simulink model "QuadrotorSimulink"  (Simulink 7.2)
settings: Solver=ode45  StartTime=0.0  StopTime=10  RelTol=1e-3
undefined symbols (not defined in the file or in its folder): Quad
settings Model: Creator=test  LastModifiedBy=test

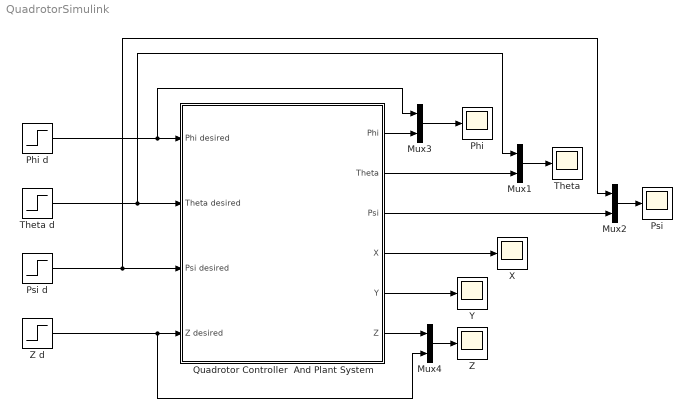
== system QuadrotorSimulink ==
  Mux{1..4} (4 alike) : Mux  Inputs=2
  Phi : Scope
  Phi d : Step  After=0  SampleTime=0
  Psi : Scope
      settings: SaveName=ScopeData2
  Psi d : Step  After=0  SampleTime=0
  Quadrotor Controller  And Plant System : Subsystem
  Theta : Scope
  Theta d : Step  After=0  SampleTime=0
  X : Scope
      settings: SaveName=ScopeData5
  Y : Scope
      settings: SaveName=ScopeData4
  Z : Scope
      settings: SaveName=ScopeData3
  Z d : Step  After=-1  SampleTime=0
  wires:
  Phi d/1 -> Quadrotor Controller  And Plant System/1(Phi desired), Mux3/1
  Theta d/1 -> Quadrotor Controller  And Plant System/2(Theta desired), Mux1/1
  Psi d/1 -> Quadrotor Controller  And Plant System/3(Psi desired), Mux2/1
  Z d/1 -> Quadrotor Controller  And Plant System/4(Z desired), Mux4/2
  Quadrotor Controller  And Plant System/1(Phi) -> Mux3/2
  Mux3/1 -> Phi/1
  Mux1/1 -> Theta/1
  Mux2/1 -> Psi/1
  Quadrotor Controller  And Plant System/2(Theta) -> Mux1/2
  Quadrotor Controller  And Plant System/3(Psi) -> Mux2/2
  Mux4/1 -> Z/1
  Quadrotor Controller  And Plant System/6(Z) -> Mux4/1
  Quadrotor Controller  And Plant System/5(Y) -> Y/1
  Quadrotor Controller  And Plant System/4(X) -> X/1

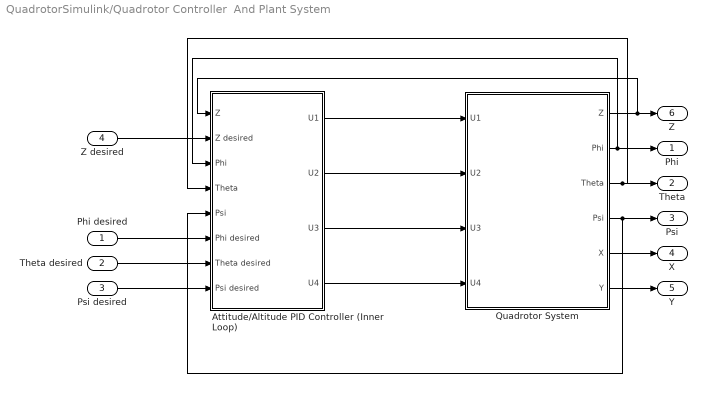
== system QuadrotorSimulink/Quadrotor Controller  And Plant System ==
  Phi desired : Inport  OutDataType=fixdt(1, 16)  OutScaling=2^0
  Theta desired : Inport  Port=2  OutDataType=fixdt(1, 16)  OutScaling=2^0
  Psi desired : Inport  Port=3  OutDataType=fixdt(1, 16)  OutScaling=2^0
  Z desired : Inport  Port=4  OutDataType=fixdt(1, 16)  OutScaling=2^0
  Attitude/Altitude PID Controller (Inner Loop) : Subsystem
  Quadrotor System : Subsystem
  Phi : Outport  OutDataType=fixdt(1, 16)  OutScaling=2^0
  Theta : Outport  Port=2  OutDataType=fixdt(1, 16)  OutScaling=2^0
  Psi : Outport  Port=3  OutDataType=fixdt(1, 16)  OutScaling=2^0
  X : Outport  Port=4  OutDataType=fixdt(1, 16)  OutScaling=2^0
  Y : Outport  Port=5  OutDataType=fixdt(1, 16)  OutScaling=2^0
  Z : Outport  Port=6  OutDataType=fixdt(1, 16)  OutScaling=2^0
  wires:
  Attitude/Altitude PID Controller (Inner Loop)/2(U2) -> Quadrotor System/2(U2)
  Psi desired/1 -> Attitude/Altitude PID Controller (Inner Loop)/8(Psi desired)
  Z desired/1 -> Attitude/Altitude PID Controller (Inner Loop)/2(Z desired)
  Attitude/Altitude PID Controller (Inner Loop)/3(U3) -> Quadrotor System/3(U3)
  Theta desired/1 -> Attitude/Altitude PID Controller (Inner Loop)/7(Theta desired)
  Phi desired/1 -> Attitude/Altitude PID Controller (Inner Loop)/6(Phi desired)
  Quadrotor System/2(Phi) -> Attitude/Altitude PID Controller (Inner Loop)/3(Phi), Phi/1
  Quadrotor System/3(Theta) -> Attitude/Altitude PID Controller (Inner Loop)/4(Theta), Theta/1
  Quadrotor System/4(Psi) -> Attitude/Altitude PID Controller (Inner Loop)/5(Psi), Psi/1
  Quadrotor System/5(X) -> X/1
  Quadrotor System/6(Y) -> Y/1
  Quadrotor System/1(Z) -> Z/1, Attitude/Altitude PID Controller (Inner Loop)/1(Z)
  Attitude/Altitude PID Controller (Inner Loop)/4(U4) -> Quadrotor System/4(U4)
  Attitude/Altitude PID Controller (Inner Loop)/1(U1) -> Quadrotor System/1(U1)

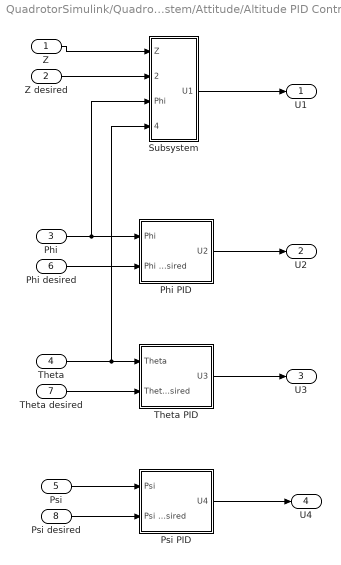
== system QuadrotorSimulink/Quadrotor Controller  And Plant System/Attitude/Altitude PID Controller (Inner Loop) ==
  Z : Inport  OutDataType=fixdt(1, 16)  OutScaling=2^0
  Z desired : Inport  Port=2  OutDataType=fixdt(1, 16)  OutScaling=2^0
  Phi : Inport  Port=3  OutDataType=fixdt(1, 16)  OutScaling=2^0
  Theta : Inport  Port=4  OutDataType=fixdt(1, 16)  OutScaling=2^0
  Psi : Inport  Port=5  OutDataType=fixdt(1, 16)  OutScaling=2^0
  Phi desired : Inport  Port=6  OutDataType=fixdt(1, 16)  OutScaling=2^0
  Theta desired : Inport  Port=7  OutDataType=fixdt(1, 16)  OutScaling=2^0
  Psi desired : Inport  Port=8  OutDataType=fixdt(1, 16)  OutScaling=2^0
  Phi PID : Subsystem
  Psi PID : Subsystem
  Subsystem : Subsystem
  Theta PID : Subsystem
  U1 : Outport  OutDataType=fixdt(1, 16)  OutScaling=2^0
  U2 : Outport  Port=2  OutDataType=fixdt(1, 16)  OutScaling=2^0
  U3 : Outport  Port=3  OutDataType=fixdt(1, 16)  OutScaling=2^0
  U4 : Outport  Port=4  OutDataType=fixdt(1, 16)  OutScaling=2^0
  wires:
  Subsystem/1(U1) -> U1/1
  Z desired/1 -> Subsystem/2(Z desired)
  Z/1 -> Subsystem/1(Z)
  Phi PID/1(U2) -> U2/1
  Phi desired/1 -> Phi PID/2(Phi desired)
  Phi/1 -> Phi PID/1(Phi), Subsystem/3(Phi)
  Psi PID/1(U4) -> U4/1
  Psi desired/1 -> Psi PID/2(Psi desired)
  Psi/1 -> Psi PID/1(Psi)
  Theta PID/1(U3) -> U3/1
  Theta desired/1 -> Theta PID/2(Theta desired)
  Theta/1 -> Theta PID/1(Theta), Subsystem/4(Theta)

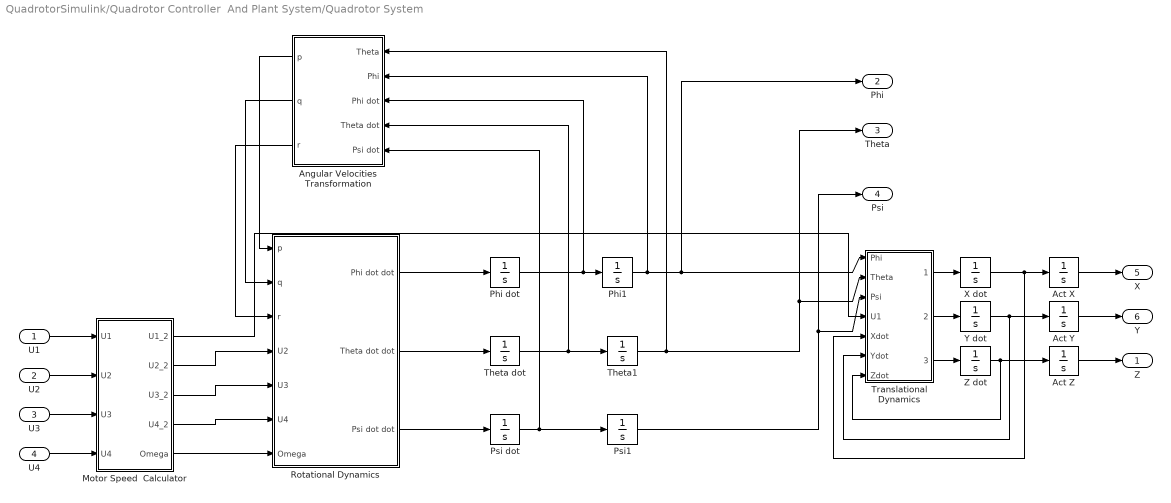
== system QuadrotorSimulink/Quadrotor Controller  And Plant System/Quadrotor System ==
  U1 : Inport  OutDataType=fixdt(1, 16)  OutScaling=2^0
  U2 : Inport  Port=2  OutDataType=fixdt(1, 16)  OutScaling=2^0
  U3 : Inport  Port=3  OutDataType=fixdt(1, 16)  OutScaling=2^0
  U4 : Inport  Port=4  OutDataType=fixdt(1, 16)  OutScaling=2^0
  Act X : Integrator
  Act Y : Integrator
  Act Z : Integrator
  Angular Velocities Transformation : Subsystem  Orientation=left
  Motor Speed  Calculator : Subsystem
  Phi dot : Integrator
  Phi1 : Integrator  ZeroCross=off
  Psi dot : Integrator  ZeroCross=off
  Psi1 : Integrator  ZeroCross=off
  Rotational Dynamics : Subsystem
  Theta dot : Integrator  ZeroCross=off
  Theta1 : Integrator  ZeroCross=off
  Translational Dynamics : Subsystem
  X dot : Integrator
  Y dot : Integrator
  Z dot : Integrator
  Z : Outport  OutDataType=fixdt(1, 16)  OutScaling=2^0
  Phi : Outport  Port=2  OutDataType=fixdt(1, 16)  OutScaling=2^0
  Theta : Outport  Port=3  OutDataType=fixdt(1, 16)  OutScaling=2^0
  Psi : Outport  Port=4  OutDataType=fixdt(1, 16)  OutScaling=2^0
  X : Outport  Port=5  OutDataType=fixdt(1, 16)  OutScaling=2^0
  Y : Outport  Port=6  OutDataType=fixdt(1, 16)  OutScaling=2^0
  wires:
  Rotational Dynamics/2(Theta dot dot) -> Theta dot/1
  Motor Speed  Calculator/5(Omega) -> Rotational Dynamics/7(Omega)
  Phi1/1 -> Translational Dynamics/1(Phi), Phi/1, Angular Velocities Transformation/2(Phi)
  Theta1/1 -> Translational Dynamics/2(Theta), Theta/1, Angular Velocities Transformation/1(Theta)
  Psi1/1 -> Translational Dynamics/3(Psi), Psi/1
  Translational Dynamics/1(x dotdot) -> X dot/1
  X dot/1 -> Act X/1, Translational Dynamics/5(Xdot)
  Y dot/1 -> Act Y/1, Translational Dynamics/6(Ydot)
  Translational Dynamics/2(y dotdot) -> Y dot/1
  Z dot/1 -> Translational Dynamics/7(Zdot), Act Z/1
  Translational Dynamics/3(z dotdot) -> Z dot/1
  Act X/1 -> X/1
  Act Y/1 -> Y/1
  Act Z/1 -> Z/1
  Psi dot/1 -> Psi1/1, Angular Velocities Transformation/5(Psi dot)
  Theta dot/1 -> Theta1/1, Angular Velocities Transformation/4(Theta dot)
  Phi dot/1 -> Phi1/1, Angular Velocities Transformation/3(Phi dot)
  Rotational Dynamics/3(Psi dot dot) -> Psi dot/1
  Rotational Dynamics/1(Phi dot dot) -> Phi dot/1
  U4/1 -> Motor Speed  Calculator/4(U4)
  U2/1 -> Motor Speed  Calculator/2(U2)
  U3/1 -> Motor Speed  Calculator/3(U3)
  Motor Speed  Calculator/2(U2_2) -> Rotational Dynamics/4(U2)
  Motor Speed  Calculator/3(U3_2) -> Rotational Dynamics/5(U3)
  Motor Speed  Calculator/1(U1_2) -> Translational Dynamics/4(U1)
  U1/1 -> Motor Speed  Calculator/1(U1)
  Motor Speed  Calculator/4(U4_2) -> Rotational Dynamics/6(U4)
  Angular Velocities Transformation/1(p) -> Rotational Dynamics/1(p)
  Angular Velocities Transformation/2(q) -> Rotational Dynamics/2(q)
  Angular Velocities Transformation/3(r) -> Rotational Dynamics/3(r)

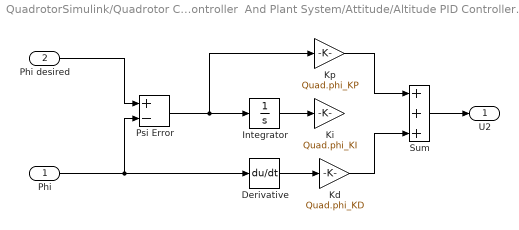
== system QuadrotorSimulink/Quadrotor Controller  And Plant System/Attitude/Altitude PID Controller (Inner Loop)/Phi PID ==
  Phi : Inport  OutDataType=fixdt(1, 16)  OutScaling=2^0
  Phi desired : Inport  Port=2  OutDataType=fixdt(1, 16)  OutScaling=2^0
  Derivative : Derivative
  Integrator : Integrator
  Kd : Gain  Gain=Quad.phi_KD  ParameterDataType=fixdt(1, 16)  ParameterScaling=2^0  OutDataType=fixdt(1, 16)  OutScaling=2^0
  Ki : Gain  Gain=Quad.phi_KI  ParameterDataType=fixdt(1, 16)  ParameterScaling=2^0  OutDataType=fixdt(1, 16)  OutScaling=2^0
  Kp : Gain  Gain=Quad.phi_KP  ParameterDataType=fixdt(1, 16)  ParameterScaling=2^0  OutDataType=fixdt(1, 16)  OutScaling=2^0
  Psi Error : Sum  Inputs=+-  OutDataType=fixdt(1, 16)  OutScaling=2^-10
  Sum : Sum  Inputs=+++  OutDataType=fixdt(1, 16)  OutScaling=2^-10
  U2 : Outport  OutDataType=fixdt(1, 16)  OutScaling=2^0
  wires:
  Phi/1 -> Psi Error/2, Derivative/1
  Phi desired/1 -> Psi Error/1
  Derivative/1 -> Kd/1
  Kp/1 -> Sum/1
  Sum/1 -> U2/1
  Psi Error/1 -> Integrator/1, Kp/1
  Integrator/1 -> Ki/1
  Kd/1 -> Sum/3

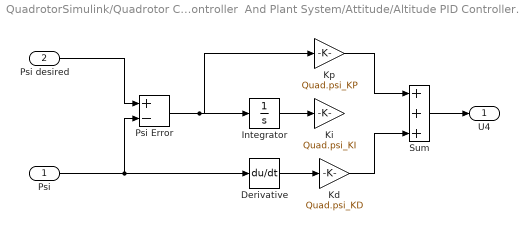
== system QuadrotorSimulink/Quadrotor Controller  And Plant System/Attitude/Altitude PID Controller (Inner Loop)/Psi PID ==
  Psi : Inport  OutDataType=fixdt(1, 16)  OutScaling=2^0
  Psi desired : Inport  Port=2  OutDataType=fixdt(1, 16)  OutScaling=2^0
  Derivative : Derivative
  Integrator : Integrator
  Kd : Gain  Gain=Quad.psi_KD  ParameterDataType=fixdt(1, 16)  ParameterScaling=2^0  OutDataType=fixdt(1, 16)  OutScaling=2^0
  Ki : Gain  Gain=Quad.psi_KI  ParameterDataType=fixdt(1, 16)  ParameterScaling=2^0  OutDataType=fixdt(1, 16)  OutScaling=2^0
  Kp : Gain  Gain=Quad.psi_KP  ParameterDataType=fixdt(1, 16)  ParameterScaling=2^0  OutDataType=fixdt(1, 16)  OutScaling=2^0
  Psi Error : Sum  Inputs=+-  OutDataType=fixdt(1, 16)  OutScaling=2^-10
  Sum : Sum  Inputs=+++  OutDataType=fixdt(1, 16)  OutScaling=2^-10
  U4 : Outport  OutDataType=fixdt(1, 16)  OutScaling=2^0
  wires:
  Psi/1 -> Psi Error/2, Derivative/1
  Psi desired/1 -> Psi Error/1
  Derivative/1 -> Kd/1
  Kp/1 -> Sum/1
  Sum/1 -> U4/1
  Psi Error/1 -> Integrator/1, Kp/1
  Integrator/1 -> Ki/1
  Kd/1 -> Sum/3

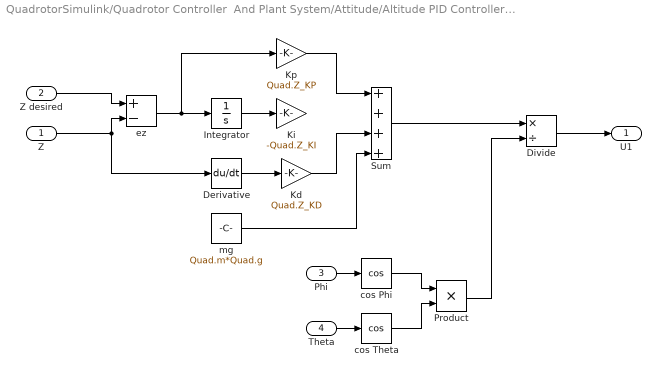
== system QuadrotorSimulink/Quadrotor Controller  And Plant System/Attitude/Altitude PID Controller (Inner Loop)/Subsystem ==
  Z : Inport  OutDataType=fixdt(1, 16)  OutScaling=2^0
  Z desired : Inport  Port=2  OutDataType=fixdt(1, 16)  OutScaling=2^0
  Phi : Inport  Port=3
  Theta : Inport  Port=4
  Derivative : Derivative
  Divide : Product  Inputs=*/  OutDataType=fixdt(1, 16)  OutScaling=2^-10
  Integrator : Integrator
  Kd : Gain  Gain=Quad.Z_KD  ParameterDataType=fixdt(1, 16)  ParameterScaling=2^0  OutDataType=fixdt(1, 16)  OutScaling=2^0
  Ki : Gain  Gain=-Quad.Z_KI  ParameterDataType=fixdt(1, 16)  ParameterScaling=2^0  OutDataType=fixdt(1, 16)  OutScaling=2^0
  Kp : Gain  Gain=Quad.Z_KP  ParameterDataType=fixdt(1, 16)  ParameterScaling=2^0  OutDataType=fixdt(1, 16)  OutScaling=2^0
  Product : Product  OutDataType=fixdt(1, 16)  OutScaling=2^0  RndMeth=Zero
  Sum : Sum  Inputs=++++  OutDataType=fixdt(1, 16)  OutScaling=2^-10
  cos Phi : Trigonometry  Operator=cos
  cos Theta : Trigonometry  Operator=cos
  ez : Sum  Inputs=+-  OutDataType=fixdt(1, 16)  OutScaling=2^-10
  mg : Constant  Value=Quad.m*Quad.g  OutDataType=fixdt(1, 16)  OutScaling=2^0
  U1 : Outport  OutDataType=fixdt(1, 16)  OutScaling=2^0
  wires:
  Z desired/1 -> ez/1
  cos Phi/1 -> Product/1
  cos Theta/1 -> Product/2
  Product/1 -> Divide/2
  Phi/1 -> cos Phi/1
  Theta/1 -> cos Theta/1
  Z/1 -> ez/2, Derivative/1
  Derivative/1 -> Kd/1
  Kp/1 -> Sum/1
  Integrator/1 -> Ki/1
  ez/1 -> Integrator/1, Kp/1
  Sum/1 -> Divide/1
  Divide/1 -> U1/1
  mg/1 -> Sum/4
  Kd/1 -> Sum/3

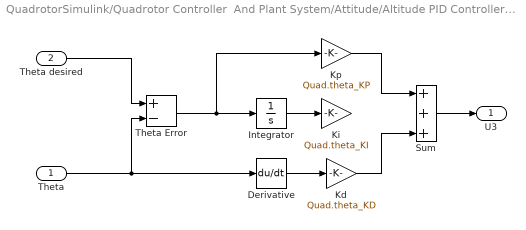
== system QuadrotorSimulink/Quadrotor Controller  And Plant System/Attitude/Altitude PID Controller (Inner Loop)/Theta PID ==
  Theta : Inport  OutDataType=fixdt(1, 16)  OutScaling=2^0
  Theta desired : Inport  Port=2  OutDataType=fixdt(1, 16)  OutScaling=2^0
  Derivative : Derivative
  Integrator : Integrator
  Kd : Gain  Gain=Quad.theta_KD  ParameterDataType=fixdt(1, 16)  ParameterScaling=2^0  OutDataType=fixdt(1, 16)  OutScaling=2^0
  Ki : Gain  Gain=Quad.theta_KI  ParameterDataType=fixdt(1, 16)  ParameterScaling=2^0  OutDataType=fixdt(1, 16)  OutScaling=2^0
  Kp : Gain  Gain=Quad.theta_KP  ParameterDataType=fixdt(1, 16)  ParameterScaling=2^0  OutDataType=fixdt(1, 16)  OutScaling=2^0
  Sum : Sum  Inputs=+++  OutDataType=fixdt(1, 16)  OutScaling=2^-10
  Theta Error : Sum  Inputs=+-  OutDataType=fixdt(1, 16)  OutScaling=2^-10
  U3 : Outport  OutDataType=fixdt(1, 16)  OutScaling=2^0
  wires:
  Theta/1 -> Theta Error/2, Derivative/1
  Theta desired/1 -> Theta Error/1
  Derivative/1 -> Kd/1
  Kp/1 -> Sum/1
  Sum/1 -> U3/1
  Theta Error/1 -> Integrator/1, Kp/1
  Integrator/1 -> Ki/1
  Kd/1 -> Sum/3

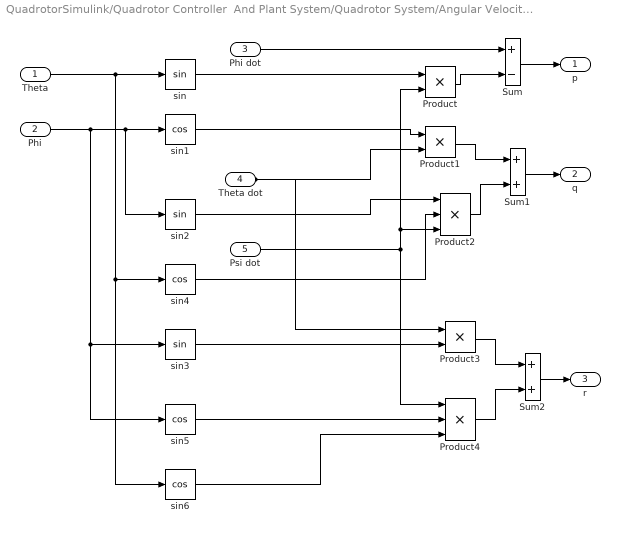
== system QuadrotorSimulink/Quadrotor Controller  And Plant System/Quadrotor System/Angular Velocities Transformation ==
  Theta : Inport  OutDataType=sfix(16)  OutScaling=2^0
  Phi : Inport  Port=2  OutDataType=sfix(16)  OutScaling=2^0
  Phi dot : Inport  Port=3  OutDataType=sfix(16)  OutScaling=2^0
  Theta dot : Inport  Port=4  OutDataType=sfix(16)  OutScaling=2^0
  Psi dot : Inport  Port=5  OutDataType=sfix(16)  OutScaling=2^0
  Product : Product  OutDataType=sfix(16)  OutScaling=2^0  RndMeth=Zero
  Product1 : Product  OutDataType=sfix(16)  OutScaling=2^0  RndMeth=Zero
  Product2 : Product  Inputs=3  OutDataType=sfix(16)  OutScaling=2^0  RndMeth=Zero
  Product3 : Product  OutDataType=sfix(16)  OutScaling=2^0  RndMeth=Zero
  Product4 : Product  Inputs=3  OutDataType=sfix(16)  OutScaling=2^0  RndMeth=Zero
  Sum : Sum  Inputs=+-  OutDataType=sfix(16)  OutScaling=2^0
  Sum1 : Sum  OutDataType=sfix(16)  OutScaling=2^0
  Sum2 : Sum  OutDataType=sfix(16)  OutScaling=2^0
  sin : Trigonometry
  sin{1,4..6} (4 alike) : Trigonometry  Operator=cos
  sin2 : Trigonometry
  sin3 : Trigonometry
  p : Outport  OutDataType=sfix(16)  OutScaling=2^0
  q : Outport  Port=2  OutDataType=sfix(16)  OutScaling=2^0
  r : Outport  Port=3  OutDataType=sfix(16)  OutScaling=2^0
  wires:
  Phi dot/1 -> Sum/1
  Theta/1 -> sin4/1, sin6/1, sin/1
  sin/1 -> Product/1
  Psi dot/1 -> Product/2, Product2/3, Product4/1
  Product/1 -> Sum/2
  Sum/1 -> p/1
  Phi/1 -> sin1/1, sin2/1, sin3/1, sin5/1
  sin1/1 -> Product1/1
  Theta dot/1 -> Product1/2, Product3/1
  Product1/1 -> Sum1/1
  sin2/1 -> Product2/1
  sin4/1 -> Product2/2
  Product2/1 -> Sum1/2
  Sum1/1 -> q/1
  sin3/1 -> Product3/2
  sin5/1 -> Product4/2
  sin6/1 -> Product4/3
  Product3/1 -> Sum2/1
  Product4/1 -> Sum2/2
  Sum2/1 -> r/1

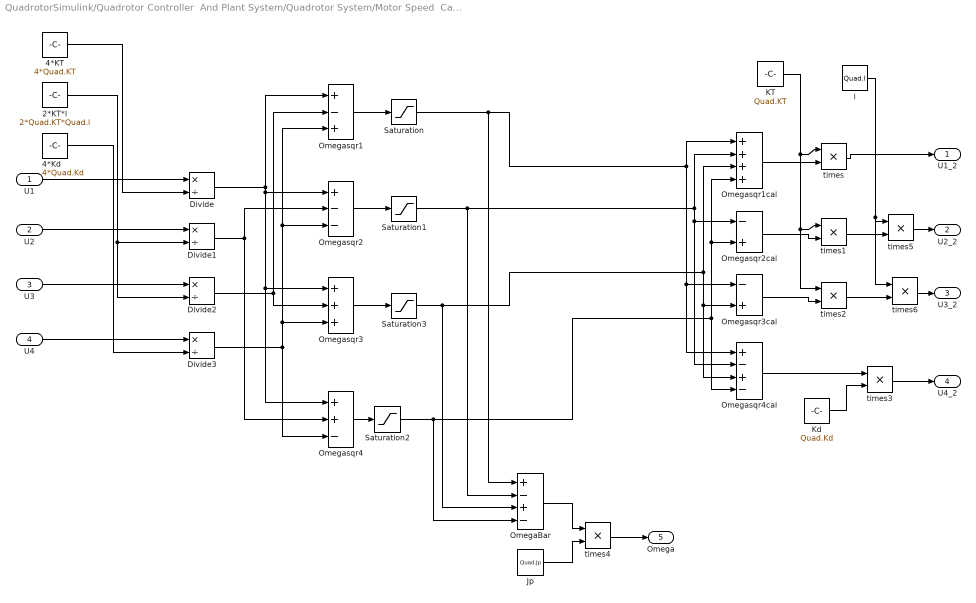
== system QuadrotorSimulink/Quadrotor Controller  And Plant System/Quadrotor System/Motor Speed  Calculator ==
  U1 : Inport  OutDataType=fixdt(1, 16)  OutScaling=2^0
  U2 : Inport  Port=2  OutDataType=fixdt(1, 16)  OutScaling=2^0
  U3 : Inport  Port=3  OutDataType=fixdt(1, 16)  OutScaling=2^0
  U4 : Inport  Port=4  OutDataType=fixdt(1, 16)  OutScaling=2^0
  2*KT*l : Constant  Value=2*Quad.KT*Quad.l  OutDataType=fixdt(1, 16)  OutScaling=2^0
  4*KT : Constant  Value=4*Quad.KT  OutDataType=fixdt(1, 16)  OutScaling=2^0
  4*Kd : Constant  Value=4*Quad.Kd  OutDataType=fixdt(1, 16)  OutScaling=2^0
  Divide{,1..3} (4 alike) : Product  Inputs=*/  OutDataType=fixdt(1, 16)  OutScaling=2^-10
  Jp : Constant  Value=Quad.Jp  OutDataType=fixdt(1, 16)  OutScaling=2^0
  KT : Constant  Value=Quad.KT  OutDataType=fixdt(1, 16)  OutScaling=2^0
  Kd : Constant  Value=Quad.Kd  OutDataType=fixdt(1, 16)  OutScaling=2^0
  OmegaBar : Sum  Inputs=+-+-  OutDataType=fixdt(1, 16)  OutScaling=2^-10
  Omegasqr1 : Sum  Inputs=+-+  OutDataType=fixdt(1, 16)  OutScaling=2^-10
  Omegasqr1cal : Sum  Inputs=++++  OutDataType=fixdt(1, 16)  OutScaling=2^-10
  Omegasqr2 : Sum  Inputs=+--  OutDataType=fixdt(1, 16)  OutScaling=2^-10
  Omegasqr2cal : Sum  Inputs=-+  OutDataType=fixdt(1, 16)  OutScaling=2^-10
  Omegasqr3 : Sum  Inputs=+++  OutDataType=fixdt(1, 16)  OutScaling=2^-10
  Omegasqr3cal : Sum  Inputs=-+  OutDataType=fixdt(1, 16)  OutScaling=2^-10
  Omegasqr4 : Sum  Inputs=++-  OutDataType=fixdt(1, 16)  OutScaling=2^-10
  Omegasqr4cal : Sum  Inputs=+-+-  OutDataType=fixdt(1, 16)  OutScaling=2^-10
  Saturation{,1..3} (4 alike) : Saturate  UpperLimit=Quad.max_motor_speed  LowerLimit=Quad.min_motor_speed  OutDataType=sfix(16)  OutScaling=2^0
  l : Constant  Value=Quad.l  OutDataType=fixdt(1, 16)  OutScaling=2^0
  times{,1..6} (7 alike) : Product  Inputs=**  OutDataType=fixdt(1, 16)  OutScaling=2^-10
  U1_2 : Outport  OutDataType=fixdt(1, 16)  OutScaling=2^0
  U2_2 : Outport  Port=2  OutDataType=fixdt(1, 16)  OutScaling=2^0
  U3_2 : Outport  Port=3  OutDataType=fixdt(1, 16)  OutScaling=2^0
  U4_2 : Outport  Port=4  OutDataType=fixdt(1, 16)  OutScaling=2^0
  Omega : Outport  Port=5  OutDataType=fixdt(1, 16)  OutScaling=2^0
  wires:
  U1/1 -> Divide/1
  4*KT/1 -> Divide/2
  U2/1 -> Divide1/1
  2*KT*l/1 -> Divide1/2, Divide2/2
  U3/1 -> Divide2/1
  U4/1 -> Divide3/1
  4*Kd/1 -> Divide3/2
  Divide/1 -> Omegasqr1/1, Omegasqr2/1, Omegasqr3/1, Omegasqr4/1
  Divide2/1 -> Omegasqr1/2, Omegasqr3/2
  Divide3/1 -> Omegasqr1/3, Omegasqr2/3, Omegasqr3/3, Omegasqr4/3
  Divide1/1 -> Omegasqr2/2, Omegasqr4/2
  OmegaBar/1 -> times4/1
  times4/1 -> Omega/1
  KT/1 -> times/1, times1/1, times2/1
  Omegasqr1cal/1 -> times/2
  Omegasqr2cal/1 -> times1/2
  Omegasqr3cal/1 -> times2/2
  Omegasqr4cal/1 -> times3/1
  Kd/1 -> times3/2
  times/1 -> U1_2/1
  times3/1 -> U4_2/1
  Jp/1 -> times4/2
  times5/1 -> U2_2/1
  times6/1 -> U3_2/1
  l/1 -> times5/1, times6/1
  times1/1 -> times5/2
  times2/1 -> times6/2
  Saturation/1 -> OmegaBar/1, Omegasqr1cal/1, Omegasqr3cal/1, Omegasqr4cal/1
  Saturation2/1 -> OmegaBar/4, Omegasqr1cal/4, Omegasqr2cal/2, Omegasqr4cal/4
  Saturation3/1 -> OmegaBar/3, Omegasqr1cal/3, Omegasqr3cal/2, Omegasqr4cal/3
  Saturation1/1 -> OmegaBar/2, Omegasqr1cal/2, Omegasqr2cal/1, Omegasqr4cal/2
  Omegasqr1/1 -> Saturation/1
  Omegasqr2/1 -> Saturation1/1
  Omegasqr3/1 -> Saturation3/1
  Omegasqr4/1 -> Saturation2/1

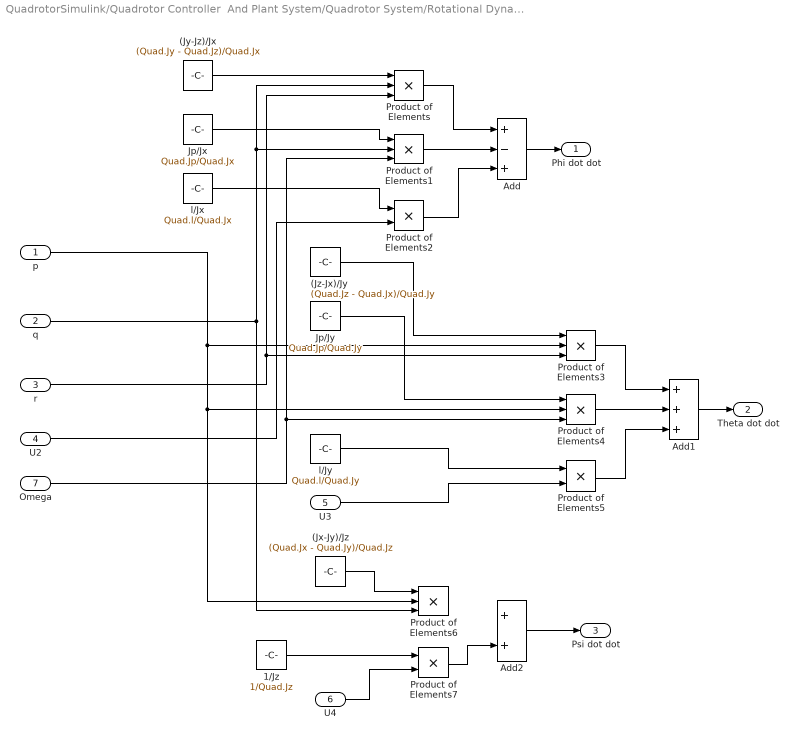
== system QuadrotorSimulink/Quadrotor Controller  And Plant System/Quadrotor System/Rotational Dynamics ==
  p : Inport  OutDataType=fixdt(1, 16)  OutScaling=2^0
  q : Inport  Port=2  OutDataType=fixdt(1, 16)  OutScaling=2^0
  r : Inport  Port=3  OutDataType=fixdt(1, 16)  OutScaling=2^0
  U2 : Inport  Port=4  OutDataType=fixdt(1, 16)  OutScaling=2^0
  U3 : Inport  Port=5  OutDataType=fixdt(1, 16)  OutScaling=2^0
  U4 : Inport  Port=6  OutDataType=fixdt(1, 16)  OutScaling=2^0
  Omega : Inport  Port=7  OutDataType=fixdt(1, 16)  OutScaling=2^0
  (Jx-Jy)/Jz : Constant  Value=(Quad.Jx - Quad.Jy)/Quad.Jz  OutDataType=fixdt(1, 16)  OutScaling=2^0
  (Jy-Jz)/Jx : Constant  Value=(Quad.Jy - Quad.Jz)/Quad.Jx  OutDataType=fixdt(1, 16)  OutScaling=2^0
  (Jz-Jx)/Jy : Constant  Value=(Quad.Jz - Quad.Jx)/Quad.Jy  OutDataType=fixdt(1, 16)  OutScaling=2^0
  1/Jz : Constant  Value=1/Quad.Jz  OutDataType=fixdt(1, 16)  OutScaling=2^0
  Add : Sum  Inputs=+-+  OutDataType=fixdt(1, 16)  OutScaling=2^-10
  Add1 : Sum  Inputs=+++  OutDataType=fixdt(1, 16)  OutScaling=2^-10
  Add2 : Sum  OutDataType=fixdt(1, 16)  OutScaling=2^-10
  Jp/Jx : Constant  Value=Quad.Jp/Quad.Jx  OutDataType=fixdt(1, 16)  OutScaling=2^0
  Jp/Jy : Constant  Value=Quad.Jp/Quad.Jy  OutDataType=fixdt(1, 16)  OutScaling=2^0
  Product of Elements{,1,3..4,6} (5 alike) : Product  Inputs=3  OutDataType=fixdt(1, 16)  OutScaling=2^-10
  Product of Elements2 : Product  OutDataType=fixdt(1, 16)  OutScaling=2^-10
  Product of Elements5 : Product  OutDataType=fixdt(1, 16)  OutScaling=2^-10
  Product of Elements7 : Product  OutDataType=fixdt(1, 16)  OutScaling=2^-10
  l/Jx : Constant  Value=Quad.l/Quad.Jx  OutDataType=fixdt(1, 16)  OutScaling=2^0
  l/Jy : Constant  Value=Quad.l/Quad.Jy  OutDataType=fixdt(1, 16)  OutScaling=2^0
  Phi dot dot : Outport  OutDataType=fixdt(1, 16)  OutScaling=2^0
  Theta dot dot : Outport  Port=2  OutDataType=fixdt(1, 16)  OutScaling=2^0
  Psi dot dot : Outport  Port=3  OutDataType=fixdt(1, 16)  OutScaling=2^0
  wires:
  Product of Elements/1 -> Add/1
  Product of Elements1/1 -> Add/2
  Product of Elements2/1 -> Add/3
  Add/1 -> Phi dot dot/1
  (Jy-Jz)/Jx/1 -> Product of Elements/1
  q/1 -> Product of Elements/2, Product of Elements1/2, Product of Elements6/3
  r/1 -> Product of Elements/3, Product of Elements3/3
  Jp/Jx/1 -> Product of Elements1/1
  l/Jx/1 -> Product of Elements2/1
  U2/1 -> Product of Elements2/2
  Omega/1 -> Product of Elements1/3, Product of Elements4/3
  Product of Elements3/1 -> Add1/1
  Product of Elements4/1 -> Add1/2
  Product of Elements5/1 -> Add1/3
  Add1/1 -> Theta dot dot/1
  (Jz-Jx)/Jy/1 -> Product of Elements3/1
  Jp/Jy/1 -> Product of Elements4/1
  l/Jy/1 -> Product of Elements5/1
  U3/1 -> Product of Elements5/2
  p/1 -> Product of Elements3/2, Product of Elements4/2, Product of Elements6/2
  Product of Elements7/1 -> Add2/2
  Add2/1 -> Psi dot dot/1
  U4/1 -> Product of Elements7/2
  1/Jz/1 -> Product of Elements7/1
  (Jx-Jy)/Jz/1 -> Product of Elements6/1

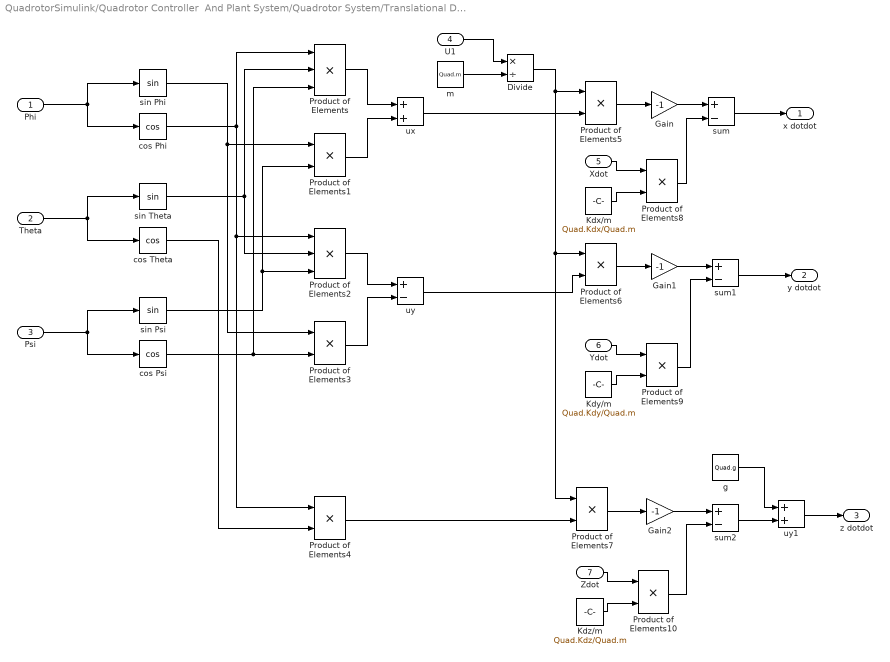
== system QuadrotorSimulink/Quadrotor Controller  And Plant System/Quadrotor System/Translational Dynamics ==
  Phi : Inport  OutDataType=fixdt(1, 16)  OutScaling=2^0
  Theta : Inport  Port=2  OutDataType=fixdt(1, 16)  OutScaling=2^0
  Psi : Inport  Port=3  OutDataType=fixdt(1, 16)  OutScaling=2^0
  U1 : Inport  Port=4  OutDataType=fixdt(1, 16)  OutScaling=2^0
  Xdot : Inport  Port=5  OutDataType=fixdt(1, 16)  OutScaling=2^0
  Ydot : Inport  Port=6  OutDataType=fixdt(1, 16)  OutScaling=2^0
  Zdot : Inport  Port=7  OutDataType=fixdt(1, 16)  OutScaling=2^0
  Divide : Product  Inputs=*/  OutDataType=fixdt(1, 16)  OutScaling=2^-10
  Gain : Gain  Gain=-1  ParameterDataType=sfix(16)  ParameterScaling=2^0  OutDataType=sfix(16)  OutScaling=2^0
  Gain1 : Gain  Gain=-1  ParameterDataType=sfix(16)  ParameterScaling=2^0  OutDataType=sfix(16)  OutScaling=2^0
  Gain2 : Gain  Gain=-1  ParameterDataType=sfix(16)  ParameterScaling=2^0  OutDataType=sfix(16)  OutScaling=2^0
  Kdx/m : Constant  Value=Quad.Kdx/Quad.m  OutDataType=fixdt(1, 16)  OutScaling=2^0
  Kdy/m : Constant  Value=Quad.Kdy/Quad.m  OutDataType=fixdt(1, 16)  OutScaling=2^0
  Kdz/m : Constant  Value=Quad.Kdz/Quad.m  OutDataType=fixdt(1, 16)  OutScaling=2^0
  Product of Elements : Product  Inputs=3  OutDataType=fixdt(1, 16)  OutScaling=2^-10
  Product of Elements{1,3..10} (9 alike) : Product  OutDataType=fixdt(1, 16)  OutScaling=2^-10
  Product of Elements2 : Product  Inputs=3  OutDataType=fixdt(1, 16)  OutScaling=2^-10
  cos Phi : Trigonometry  Operator=cos
  cos Psi : Trigonometry  Operator=cos
  cos Theta : Trigonometry  Operator=cos
  g : Constant  Value=Quad.g  OutDataType=fixdt(1, 16)  OutScaling=2^0
  m : Constant  Value=Quad.m  OutDataType=fixdt(1, 16)  OutScaling=2^0
  sin Phi : Trigonometry
  sin Psi : Trigonometry
  sin Theta : Trigonometry
  sum : Sum  Inputs=+-  OutDataType=fixdt(1, 16)  OutScaling=2^-10
  sum1 : Sum  Inputs=+-  OutDataType=fixdt(1, 16)  OutScaling=2^-10
  sum2 : Sum  Inputs=+-  OutDataType=fixdt(1, 16)  OutScaling=2^-10
  ux : Sum  OutDataType=fixdt(1, 16)  OutScaling=2^-10
  uy : Sum  Inputs=+-  OutDataType=fixdt(1, 16)  OutScaling=2^-10
  uy1 : Sum  OutDataType=fixdt(1, 16)  OutScaling=2^-10
  x dotdot : Outport  OutDataType=fixdt(1, 16)  OutScaling=2^0
  y dotdot : Outport  Port=2  OutDataType=fixdt(1, 16)  OutScaling=2^0
  z dotdot : Outport  Port=3  OutDataType=fixdt(1, 16)  OutScaling=2^0
  wires:
  Phi/1 -> sin Phi/1, cos Phi/1
  Theta/1 -> sin Theta/1, cos Theta/1
  Psi/1 -> sin Psi/1, cos Psi/1
  sin Theta/1 -> Product of Elements/2, Product of Elements2/2
  cos Psi/1 -> Product of Elements/3, Product of Elements3/2
  cos Phi/1 -> Product of Elements/1, Product of Elements2/1, Product of Elements4/1
  sin Phi/1 -> Product of Elements1/1, Product of Elements3/1
  sin Psi/1 -> Product of Elements1/2, Product of Elements2/3
  Product of Elements/1 -> ux/1
  Product of Elements1/1 -> ux/2
  ux/1 -> Product of Elements5/2
  Product of Elements2/1 -> uy/1
  Product of Elements3/1 -> uy/2
  uy/1 -> Product of Elements6/2
  cos Theta/1 -> Product of Elements4/2
  Product of Elements4/1 -> Product of Elements7/2
  U1/1 -> Divide/1
  m/1 -> Divide/2
  Divide/1 -> Product of Elements5/1, Product of Elements6/1, Product of Elements7/1
  uy1/1 -> z dotdot/1
  Product of Elements5/1 -> Gain/1
  Product of Elements6/1 -> Gain1/1
  Xdot/1 -> Product of Elements8/1
  Kdx/m/1 -> Product of Elements8/2
  Gain/1 -> sum/1
  Product of Elements8/1 -> sum/2
  sum/1 -> x dotdot/1
  Ydot/1 -> Product of Elements9/1
  Kdy/m/1 -> Product of Elements9/2
  Gain1/1 -> sum1/1
  Product of Elements9/1 -> sum1/2
  sum1/1 -> y dotdot/1
  Zdot/1 -> Product of Elements10/1
  Kdz/m/1 -> Product of Elements10/2
  Gain2/1 -> sum2/1
  Product of Elements7/1 -> Gain2/1
  g/1 -> uy1/1
  sum2/1 -> uy1/2
  Product of Elements10/1 -> sum2/2
